simulink model "system_simulator"  (R2024b)
settings: Solver=FixedStepAuto  StartTime=0.0  StopTime=35  FixedStep=0.001  RelTol=1e-3
undefined symbols (not defined in the file): DiscIntNeverNeededParam
settings Model: Creator=deniz  LastModifiedBy=ashha

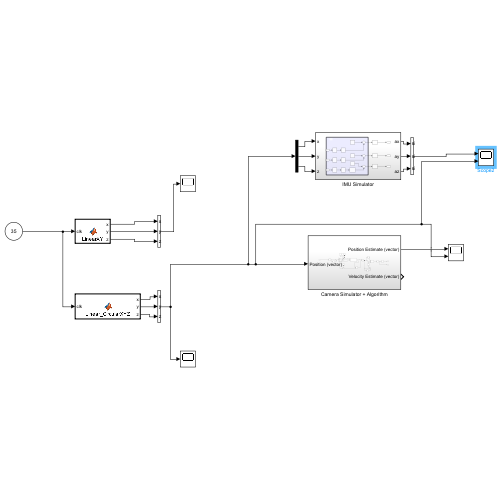
[thumbnail: Simulink's stored preview of the top-level diagram]
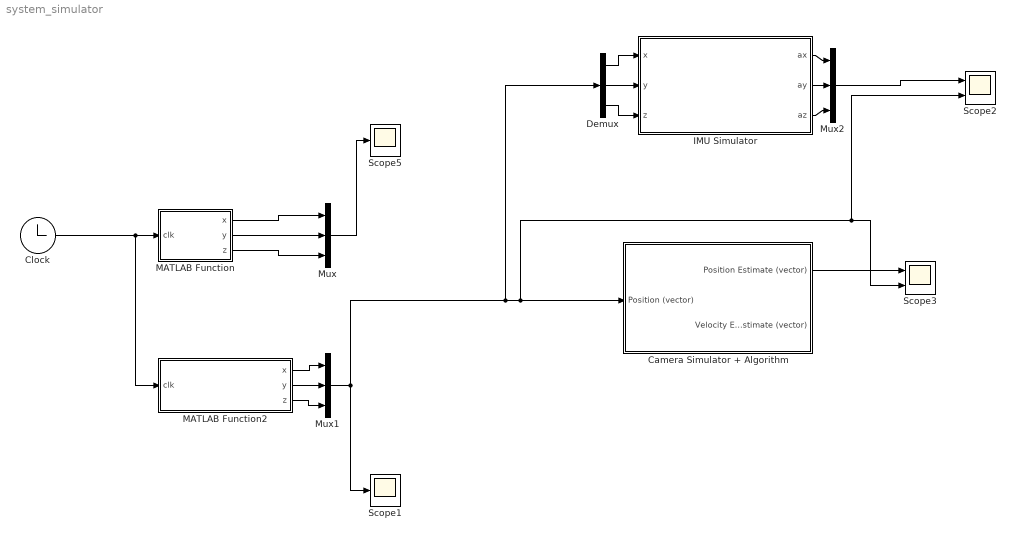
== system system_simulator ==
  Camera Simulator + Algorithm : Subsystem
  Clock : Clock
  Demux : Demux  Outputs=3
  IMU Simulator : Subsystem
  MATLAB Function : MATLAB Function  TreatAsAtomicUnit=on
  MATLAB Function2 : MATLAB Function  TreatAsAtomicUnit=on
  Mux : Mux  Inputs=3
      settings: DisplayOption=signals
  Mux1 : Mux  Inputs=3
      settings: DisplayOption=signals
  Mux2 : Mux  Inputs=3
      settings: DisplayOption=signals
  Scope1 : Scope
  Scope2 : Scope  NumInputPorts=2
  Scope3 : Scope  NumInputPorts=2
  Scope5 : Scope
  wires:
  Clock/1 -> MATLAB Function2/1(clk), MATLAB Function/1(clk)
  MATLAB Function2/2(y) -> Mux1/2
  MATLAB Function2/1(x) -> Mux1/1
  MATLAB Function2/3(z) -> Mux1/3
  Demux/1 -> IMU Simulator/1(x)
  Demux/2 -> IMU Simulator/2(y)
  Demux/3 -> IMU Simulator/3(z)
  IMU Simulator/1(ax) -> Mux2/1
  IMU Simulator/2(ay) -> Mux2/2
  IMU Simulator/3(az) -> Mux2/3
  MATLAB Function/1(x) -> Mux/1
  MATLAB Function/2(y) -> Mux/2
  MATLAB Function/3(z) -> Mux/3
  Mux/1 -> Scope5/1
  Mux2/1 -> Scope2/1
  Mux1/1 -> Scope1/1, Demux/1, Scope2/2, Scope3/2, Camera Simulator + Algorithm/1(Position (vector))
  Camera Simulator + Algorithm/1(Position Estimate (vector)) -> Scope3/1

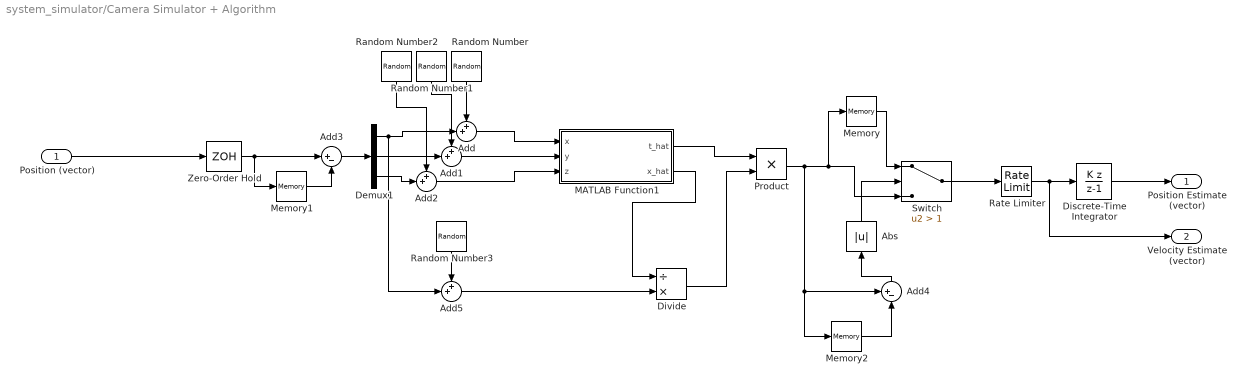
== system system_simulator/Camera Simulator + Algorithm ==
  Position (vector) : Inport
  Abs : Abs  SaturateOnIntegerOverflow=off
  Add{,1..2,5} (4 alike) : Sum  Inputs=++|
  Add3 : Sum  Inputs=|+-
  Add4 : Sum  Inputs=+-|
  Demux1 : Demux  Outputs=3
  Discrete-Time Integrator : DiscreteIntegrator  IntegratorMethod=Accumulation: Backward Euler  SampleTime=1/100  ICPrevOutput=DiscIntNeverNeededParam  ICPrevScaledInput=DiscIntNeverNeededParam
  Divide : Product  Inputs=/*
  MATLAB Function1 : MATLAB Function  TreatAsAtomicUnit=on
  Memory : Memory
  Memory1 : Memory  InheritSampleTime=on  LinearizeAsDelay=on
  Memory2 : Memory  InheritSampleTime=on  LinearizeAsDelay=on
  Product : Product
  Random Number : RandomNumber  Variance=0.01  Seed=42  SampleTime=1/100
  Random Number1 : RandomNumber  Variance=0.01  Seed=41  SampleTime=1/100
  Random Number2 : RandomNumber  Variance=0.01  Seed=49  SampleTime=1/100
  Random Number3 : RandomNumber  Variance=0.005  Seed=21  SampleTime=1/100
  Rate Limiter : RateLimiter  RisingSlewLimit=5/0.01  FallingSlewLimit=-5/0.01  SampleTimeMode=inherited
  Switch : Switch  Criteria=u2 > Threshold  Threshold=1  SaturateOnIntegerOverflow=off  InputSameDT=off
  Zero-Order Hold : ZeroOrderHold  SampleTime=1/100
  Position Estimate (vector) : Outport
  Velocity Estimate (vector) : Outport  Port=2
  wires:
  Add1/1 -> MATLAB Function1/2(y)
  Random Number2/1 -> Add2/1
  Demux1/1 -> Add5/2, Add/2
  Demux1/2 -> Add1/2
  Demux1/3 -> Add2/2
  MATLAB Function1/1(t_hat) -> Product/1
  Switch/1 -> Rate Limiter/1
  Memory2/1 -> Add4/2
  Product/1 -> Memory2/1, Add4/1, Memory/1, Switch/3
  Zero-Order Hold/1 -> Add3/1, Memory1/1
  Add/1 -> MATLAB Function1/1(x)
  MATLAB Function1/2(x_hat) -> Divide/1
  Add3/1 -> Demux1/1
  Divide/1 -> Product/2
  Random Number1/1 -> Add1/1
  Add2/1 -> MATLAB Function1/3(z)
  Add5/1 -> Divide/2
  Random Number3/1 -> Add5/1
  Memory1/1 -> Add3/2
  Memory/1 -> Switch/1
  Rate Limiter/1 -> Velocity Estimate (vector)/1, Discrete-Time Integrator/1
  Random Number/1 -> Add/1
  Add4/1 -> Abs/1
  Abs/1 -> Switch/2
  Position (vector)/1 -> Zero-Order Hold/1
  Discrete-Time Integrator/1 -> Position Estimate (vector)/1

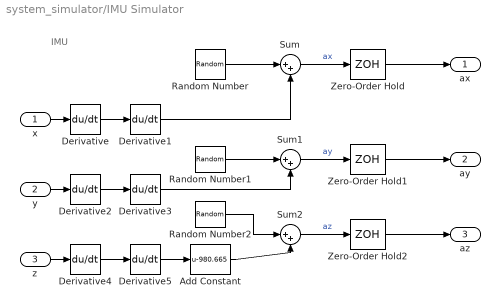
== system system_simulator/IMU Simulator ==
  note: IMU
  x : Inport
  y : Inport  Port=2
  z : Inport  Port=3
  Add Constant : Bias  Bias=-980.665  SaturateOnIntegerOverflow=off
  Derivative{,1..5} (6 alike) : Derivative
  Random Number : RandomNumber  Variance=25  Seed=42  SampleTime=0.001
  Random Number1 : RandomNumber  Variance=25  Seed=49  SampleTime=0.001
  Random Number2 : RandomNumber  Variance=25  Seed=34  SampleTime=0.001
  Sum : Sum  Inputs=|++
  Sum1 : Sum  Inputs=|++
  Sum2 : Sum  Inputs=|++
  Zero-Order Hold : ZeroOrderHold  SampleTime=1/100
  Zero-Order Hold1 : ZeroOrderHold  SampleTime=1/100
  Zero-Order Hold2 : ZeroOrderHold  SampleTime=1/100
  ax : Outport
  ay : Outport  Port=2
  az : Outport  Port=3
  wires:
  Derivative4/1 -> Derivative5/1
  Derivative2/1 -> Derivative3/1
  Derivative3/1 -> Sum1/2
  Derivative5/1 -> Add Constant/1
  Random Number1/1 -> Sum1/1
  Random Number2/1 -> Sum2/1
  y/1 -> Derivative2/1
  Sum/1 -> Zero-Order Hold/1  "ax"
  Random Number/1 -> Sum/1
  Derivative/1 -> Derivative1/1
  Add Constant/1 -> Sum2/2
  Derivative1/1 -> Sum/2
  z/1 -> Derivative4/1
  Sum2/1 -> Zero-Order Hold2/1  "az"
  Sum1/1 -> Zero-Order Hold1/1  "ay"
  x/1 -> Derivative/1
  Zero-Order Hold/1 -> ax/1
  Zero-Order Hold1/1 -> ay/1
  Zero-Order Hold2/1 -> az/1

== matlab function system_simulator/Camera Simulator + Algorithm/MATLAB Function1 ==
  data: x input; t_hat output; y input; z input; x_hat output
function [t_hat, x_hat]= EgoMotion(x, y, z)

X = [x y z]';

t_abs = sqrt(x^2 + y^2 + z^2);

t_hat = X/t_abs;
x_hat = t_hat(1);

== matlab function system_simulator/MATLAB Function ==
  data: x output; clk input; y output; z output
function [x, y, z] = LinearXY(clk)
%#codegen
% SYNTHETICPATH  Generates a 5-leg piecewise-cubic path in (x,y),
%                with constant z=180 cm.
%
% INPUT:
%   clk : scalar time from a Simulink Clock block
% OUTPUT:
%   x,y,z : scalar positions (cm)

    % --- Initialize outputs as scalars so Simulink knows they are 1x1 doubles ---
    x = 0.0;
    y = 0.0;
    z = 0.0;

    % --- Define waypoints as a cell array. Each cell is a [3x1] vector. ---
    % If codegen complains about cell arrays, see alternative "Matrix version" below.
    P = cell(6,1);
    P{1} = [0.0;    0.0;   0];
    P{2} = [-50.0;  100.0;   0];
    P{3} = [100.0; 100.0;  0];
    P{4} = [-100.0;-100.0; 0];
    P{5} = [100.0; -100.0; 0];
    P{6} = [0.0;   0.0;    0];
0
    % --- Define peak velocities for each leg, in cm/s ---
    %   (2 m/s=200 cm/s, 1=100, 3=300, 0.5=50, 1.5=150)
    Vmaxs = [200.0, 100.0, 300.0, 50.0, 150.0];

    % --- Number of legs is 5 (since we have P1..P6) ---
    nLegs = 5;

    % --- Precompute distance and time for each leg ---
    D = zeros(1,nLegs);
    T = zeros(1,nLegs);
    for i = 1:nLegs
        dVec = P{i+1}(1:2) - P{i}(1:2);  % 2D displacement (x,y)
        dist = norm(dVec);
        D(i) = dist;
        % For a 0->Vmax->0 cubic, total time T = 1.5*(dist / Vmax)
        T(i) = 1.5 * dist / Vmaxs(i);
    end

    % --- Cumulative times to identify time intervals ---
    cumT = cumsum(T);

    % If clk < 0, just hold the initial waypoint
    if clk < 0
        x = P{1}(1);
        y = P{1}(2);
        z = P{1}(3);
        return;
    end

    % --- Figure out which leg we are in based on clk ---
    legIndex = 0;
    for i = 1:nLegs
        if clk <= cumT(i)
            legIndex = i;
            break;
        end
    end

    % If we're beyond final leg, hold final position
    if legIndex == 0
        x = P{nLegs+1}(1);
        y = P{nLegs+1}(2);
        z = P{nLegs+1}(3);
        return;
    end

    % --- Local time in this leg ---
    if legIndex == 1
        tStartLeg = 0.0;
    else
        tStartLeg = cumT(legIndex-1);
    end
    localTime   = clk - tStartLeg;
    segDuration = T(legIndex);

    % --- Normalize local time s in [0..1] ---
    s = localTime / segDuration;
    if s < 0
        s = 0;
    elseif s > 1
        s = 1;
    end

    % --- Cubic blend  p(s)=3s^2 -2s^3 for smooth 0->1 with zero velocities ---
    blend = 3.0 * s^2 - 2.0 * s^3;

    % --- Interpolate between startPos and endPos in (x,y). z=180 constant. ---
    startPos = P{legIndex};
    endPos   = P{legIndex+1};

    x = startPos(1) + blend * (endPos(1) - startPos(1));
    y = startPos(2) + blend * (endPos(2) - startPos(2));
    z = 0;
end

== matlab function system_simulator/MATLAB Function2 ==
  data: x output; clk input; y output; z output
function [x, y, z] = Linear_CircularXYZ(clk)
%#codegen
% 7-SEGMENT ARC+LINE PATH WITH VARIABLE Z
%
% XY path (same as before):
%   1) Full circle center(0,0), radius=100, from (-100,0) to same point
%   2) Line (-100,0)->(0,0)
%   3) Full circle center(0,50) radius=50, from (0,0)->(0,0)
%   4) Line (0,0)->(0,-100)
%   5) Line (0,-100)->(100,100)
%   6) Half circle center(0,0) from (100,100)->(-100,-100)
%   7) Line (-100,-100)->(0,0)
%
% Meanwhile, Z transitions each segment:
%   1) 00->80  (vmax=1.0m/s =>100cm/s)
%   2) 80->50  (0.5m/s =>50cm/s)
%   3) 50->80  (1.5m/s =>150cm/s)
%   4) 80->00
%   5) 00->00
%   6) 00->80
%   7) 80->00
%
% (Adjust these as you like; the code smoothly blends X,Y,Z.)

    x=0.0; y=0.0; z=0.0; % initialize

    nSeg=7;
    typeSeg=zeros(1,nSeg); % 1=arc,2=line
    Vmax=zeros(1,nSeg);

    centerX=zeros(1,nSeg); centerY=zeros(1,nSeg); radiusVal=zeros(1,nSeg);
    thetaStart=zeros(1,nSeg); thetaEnd=zeros(1,nSeg);

    startX=zeros(1,nSeg); startY=zeros(1,nSeg);
    endX  =zeros(1,nSeg); endY  =zeros(1,nSeg);

    startZarr=zeros(1,nSeg); endZarr=zeros(1,nSeg);

    %--- Segment 1: full circle (0,0)->same
    i=1;
    typeSeg(i)=1;
    centerX(i)=50.0; centerY(i)=0.0; radiusVal(i)=50.0;
    thetaStart(i)=pi;   % -100,0 => angle=π
    thetaEnd(i)=3*pi;   % +2π => ends same place
    Vmax(i)=100.0;      % 1.0 m/s
    startZarr(i)=00.0; endZarr(i)=50.0;

    %--- Segment 2: line (0,0)->(0,0)
    i=2;
    typeSeg(i)=2;
    startX(i)=0.0; startY(i)=0.0;
    endX(i)=0.0;       endY(i)=0.0;
    Vmax(i)=50.0;      % 0.5 m/s
    startZarr(i)=50.0; endZarr(i)=50.0;

    %--- Segment 3: full circle center(0,50), radius=50
    i=3;
    typeSeg(i)=1;
    centerX(i)=0.0; centerY(i)=50.0; radiusVal(i)=50.0;
    thetaStart(i)=-pi/2;
    thetaEnd(i)=3*pi/2;
    Vmax(i)=150.0;     % 1.5 m/s
    startZarr(i)=50.0; endZarr(i)=80.0;

    %--- Segment 4: line (0,0)->(0,-100)
    i=4;
    typeSeg(i)=2;
    startX(i)=0.0; startY(i)=0.0; endX(i)=0.0; endY(i)=-100.0;
    Vmax(i)=100.0;  % 1.0 m/s
    startZarr(i)=80.0; endZarr(i)=00.0;

    %--- Segment 5: line (0,-100)->(100,100)
    i=5;
    typeSeg(i)=2;
    startX(i)=0.0; startY(i)=-100.0; endX(i)=100.0; endY(i)=100.0;
    Vmax(i)=50.0;   % 0.5 m/s
    startZarr(i)=00.0; endZarr(i)=00.0;

    %--- Segment 6: half circle (100,100)->(-100,-100) center(0,0)
    i=6;
    typeSeg(i)=1;
    centerX(i)=0.0; centerY(i)=0.0;
    radiusVal(i)=sqrt(100^2+100^2);
    thetaStart(i)=pi/4;   % 45°
    thetaEnd(i)=5*pi/4;   % 225°
    Vmax(i)=150.0;  % 1.5 m/s
    startZarr(i)=00.0; endZarr(i)=80.0;

    %--- Segment 7: line (-100,-100)->(0,0)
    i=7;
    typeSeg(i)=2;
    startX(i)=-100.0; startY(i)=-100.0;
    endX(i)=0.0;      endY(i)=0.0;
    Vmax(i)=100.0;  % 1.0 m/s
    startZarr(i)=80.0; endZarr(i)=0.0;

    %--- Compute distances (XY) & times
    D=zeros(1,nSeg);  T=zeros(1,nSeg);
    for i=1:nSeg
        if typeSeg(i)==1
            arcLen=radiusVal(i)*abs(thetaEnd(i)-thetaStart(i));
            D(i)=arcLen;
        else
            dx=endX(i)-startX(i);
            dy=endY(i)-startY(i);
            D(i)=sqrt(dx*dx+dy*dy);
        end
        T(i)=1.5*(D(i)/Vmax(i));
    end
    cumT=cumsum(T);

    %--- If clk<0, hold first
    if clk<0
        [xx,yy]=getSegmentStart(typeSeg(1), centerX(1),centerY(1),radiusVal(1),thetaStart(1),...
                                startX(1),startY(1));
        x=xx; y=yy; z=startZarr(1);
        return;
    end

    segIndex=0;
    for i=1:nSeg
        if clk<=cumT(i)
            segIndex=i;
            break;
        end
    end
    if segIndex==0
        % hold final
        [xx,yy]=getSegmentEnd(typeSeg(nSeg), centerX(nSeg),centerY(nSeg),radiusVal(nSeg),thetaEnd(nSeg),...
                              endX(nSeg),endY(nSeg));
        x=xx; y=yy; z=endZarr(nSeg);
        return;
    end

    if segIndex==1
        tStart=0.0;
    else
        tStart=cumT(segIndex-1);
    end
    localTime=clk - tStart;
    segDuration=T(segIndex);

    s=localTime/segDuration;
    if s<0, s=0; end
    if s>1, s=1; end

    blend=3*s^2 - 2*s^3;

    % X,Y
    if typeSeg(segIndex)==1
        % Arc
        th0=thetaStart(segIndex);
        th1=thetaEnd(segIndex);
        cx=centerX(segIndex);
        cy=centerY(segIndex);
        r=radiusVal(segIndex);
        th=th0 + blend*(th1 - th0);
        x=cx + r*cos(th);
        y=cy + r*sin(th);
    else
        % Line
        sx=startX(segIndex);
        sy=startY(segIndex);
        ex=endX(segIndex);
        ey=endY(segIndex);
        x=sx + blend*(ex - sx);
        y=sy + blend*(ey - sy);
    end

    % Z
    z0=startZarr(segIndex);
    z1=endZarr(segIndex);
    z = z0 + blend*(z1 - z0);
end

%---- Helpers
function [xx, yy] = getSegmentStart(typ, cx, cy, r, th0, sx, sy)
    if typ==1
        xx = cx + r*cos(th0);
        yy = cy + r*sin(th0);
    else
        xx = sx; yy = sy;
    end
end

function [xx, yy] = getSegmentEnd(typ, cx, cy, r, th1, ex, ey)
    if typ==1
        xx = cx + r*cos(th1);
        yy = cy + r*sin(th1);
    else
        xx = ex; yy = ey;
    end
end
